simulink model "lift"  (R2020b)
settings: Solver=VariableStepAuto  StartTime=0.0  StopTime=10.0  RelTol=1e-3
settings Model: Creator=Manasi  LastModifiedBy=Manasi

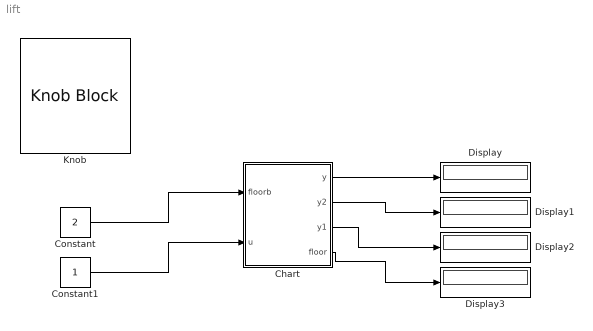
== system lift ==
  Chart : Stateflow chart  TreatAsAtomicUnit=on
  Constant : Constant  Value=2
  Constant1 : Constant
  Display{,1..3} (4 alike) : Display
  Knob : KnobBlock  ScaleMax=5  TickInterval=1
  wires:
  Chart/1(y) -> Display/1
  Chart/2(y2) -> Display1/1
  Chart/3(y1) -> Display2/1
  Chart/4(floor) -> Display3/1
  Constant/1 -> Chart/1(floorb)
  Constant1/1 -> Chart/2(u)

== stateflow chart lift/Chart ==
  state Elevator_on
    entry: y=1;
    note: [floorb<floor]{y1= 1 }
    state DOWN
      entry:
      floor=floor-1;
    state Delay1
      entry:
      floor=floor-1;
    state Idle_state
      entry: y1=0;
    state UP
      entry:
      floor=floor+1;
    state Delay
      entry:
      floor=floor+1;
    state Door_open1
      entry:
      y2=1;
    state Door_close1
      entry:
      y2=0;
    state Door_open
      entry:
      y2=1;
    state Door_close
      entry:
      y2=0;
    (default) -> Idle_state
    DOWN -> Delay1 [order 1] : [floorb<floor]
    Idle_state -> DOWN [order 2]
    Delay1 -> DOWN [order 1] : [floorb<floor]
    Idle_state -> UP [order 1] : [floorb>floor]{y1=1}
    DOWN -> Door_open1 [order 2] : [floorb==floor]
    Delay1 -> Door_open1 [order 2] : [floor==floorb]
    Delay -> UP [order 1] : [floorb>floor]
    UP -> Delay [order 1] : [floorb>floor]
    Door_open1 -> Door_close1 : [after(5,sec)]
    UP -> Door_open [order 2] : [floorb==floor]
    Delay -> Door_open [order 2] : [floor==floorb]
    Door_open -> Door_close : [after(5,sec)]
  state Elevator_off
    entry: y=0;
  (default) -> Elevator_on
  Elevator_on -> Elevator_off : [u==0]
  Elevator_off -> Elevator_on : [u==1]
  data: floorb input [0..5]; u input; y output [0..1]; y2 output [0..1]; y1 output [0..1]; floor output [0..5] =0
